simulink model "GenererLaSource1"  (R2020a)
settings: Solver=FixedStepDiscrete  StartTime=0.0  StopTime=0.001  RelTol=1e-3
libraries: commrandsrc2 x1
settings Model: Creator=Vincent  LastModifiedBy=J-MENTION
settings DataIOCC: LimitDataPoints=on  SaveFormat=Array  SignalLoggingSaveFormat=ModelDataLogs  ReturnWorkspaceOutputs=off
settings OptimizationCC: ExpressionDepthLimit=2147483647  LifeSpan=inf
settings DebuggingCC: UnderspecifiedInitializationDetection=Classic  MergeDetectMultiDrivingBlocksExec=none  SolverPrmCheckMsg=warning  FcnCallInpInsideContextMsg=warning  StateNameClashWarn=warning  SFUnexpectedBacktrackingDiag=warning  SFNoUnconditionalDefaultTransitionDiag=warning  SFExecutionAtInitializationDiag=none  ArithmeticOperatorsInVariantConditions=warning
settings HardwareCC: ProdBitPerPointer=32  ProdBitPerSizeT=32  ProdBitPerPtrDiffT=32  ProdLargestAtomicFloat=None  ProdIntDivRoundTo=Undefined  ProdEndianess=Unspecified  ProdWordSize=32  ProdHWDeviceType=32-bit Generic
settings ModelReferenceCC: PropagateSignalLabelsOutOfModel=off
settings SFSimCC: SimUseLocalCustomCode=off  CustomCodeUndefinedFunction=UseInterfaceOnly
settings RTWCC: RTWUseLocalCustomCode=off
settings CodeAppCC: StateflowObjectComments=on
settings GRTTargetCC: TargetLangStandard=C89/C90 (ANSI)  CombineOutputUpdateFcns=off  GRTInterface=on
settings ConfigComp: CovMetricSettings=dw  CovHtmlReporting=on  CovSaveCumulativeToWorkspaceVar=on  CovSaveSingleToWorkspaceVar=on  CovExternalEMLEnable=off

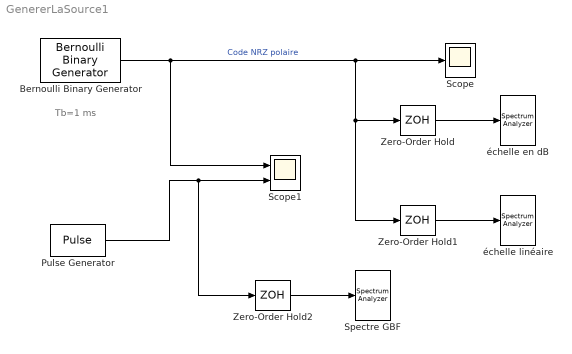
== system GenererLaSource1 ==
  note: Tb=1 ms
  Bernoulli Binary Generator : commrandsrc2/Bernoulli Binary Generator  P=0.5  seed=61  Ts=1e-3  frameBased=off  sampPerFrame=1  orient=off  outDataType=double
      settings: SourceProductBaseCode=CM
  Pulse Generator : DiscretePulseGenerator  Period=10  PulseWidth=5  SampleTime=1/5000
  Scope : Scope
  Scope1 : Scope  NumInputPorts=2
  "Spectre GBF " : SpectrumAnalyzer
  Zero-Order Hold : ZeroOrderHold  SampleTime=1/10000
  Zero-Order Hold1 : ZeroOrderHold  SampleTime=1/10000
  Zero-Order Hold2 : ZeroOrderHold  SampleTime=1/10000
  échelle en dB : SpectrumAnalyzer
  échelle linéaire : SpectrumAnalyzer
  wires:
  Bernoulli Binary Generator/1 -> Scope1/1, Scope/1, Zero-Order Hold/1, Zero-Order Hold1/1  "Code NRZ polaire"
  Zero-Order Hold/1 -> échelle en dB/1
  Zero-Order Hold1/1 -> échelle linéaire/1
  Pulse Generator/1 -> Zero-Order Hold2/1, Scope1/2
  Zero-Order Hold2/1 -> "Spectre GBF "/1
